simulink model "hodumaru"  (R2023a)
settings: Solver=VariableStepAuto  StartTime=0.0  StopTime=10.0  RelTol=1e-3
undefined symbols (not defined in the file): _NA, Addr, Control, DFSW, DSFW, Kill, NeuralCodedData, R_EN, RC, RC_FINAL, Spike
(part 1 of 2)
settings Model: Creator=user  LastModifiedBy=x1t2

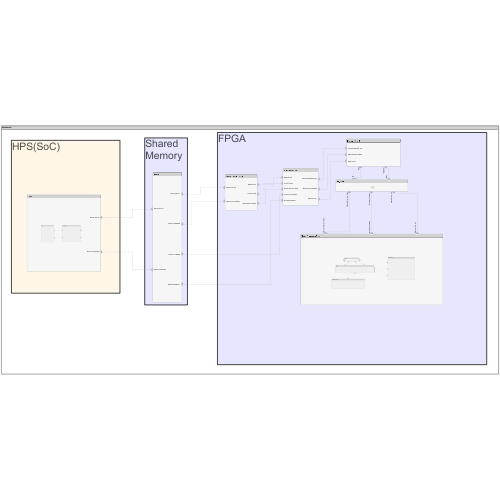
[thumbnail: Simulink's stored preview of the top-level diagram]
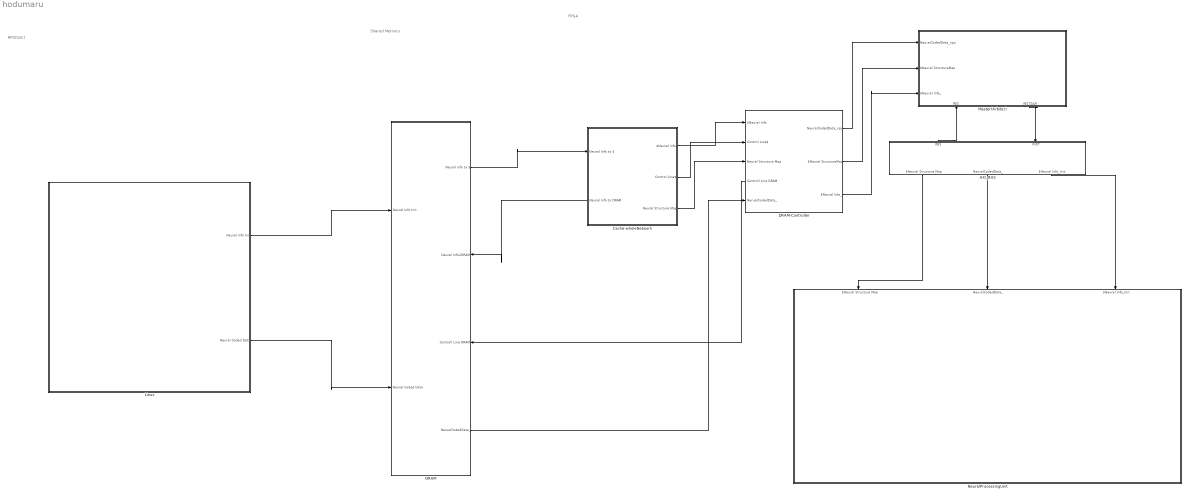
== system hodumaru ==
  note: Shared
      | Memory
  note: HPS(SoC)
  note: FPGA
  AXI_BUS : Subsystem
      settings: PortSchema="{\"entries\":[{\"content\":{\"headerSize\":26,\"margin\":15,\"minimumSpacing\":25,\"sides\":[{\"content\":{},\"type\":\"ConnectorPlacement.EquallySpacedRectSide\",\"uuid\":\"08b5c2e0-5e4b-4108-9213-5cb3cfbc2fc7\"},{\"content\":{\"side\":\"RIGHT\"},\"type\":\"ConnectorPlacement.EquallySpacedRectSide\",\"uuid\":\"cef344b6-f3e5-417a-912f-da0044eb54ca\"},{\"content\":{\"connectorIds\":[\"Out3\",\"In1\"],\"side\":\"TOP\"},\"type\":\"ConnectorPlacement.EquallySpacedRectSide\",\"uuid\":\"0b83641f-e918-4d2c-8db0-09bb563129af\"},{\"content\":{\"connectorIds\":[\"Out1\",\"Out2\",\"Out4\"],\"side\":\"BOTTOM\"},\"type\":\"ConnectorPlacement.EquallySpacedRectSide\",\"uuid\":\"7ad7297b-5e88-44bc-b04f-1700d4001bfc\"}]},\"type\":\"ConnectorPlacement.EquallySpacedConnector\",\"uuid\":\"45bfd962-fc80-412c-925f-742c48c6b5c0\"}],\"packageUris\":[\"http://schema.mathworks.com/mf0/Connector/R2020b\"],\"version\":\"1.0\"}"
  Cache-wholeNetwork : Subsystem
      settings: PortSchema="{\"entries\":[{\"content\":{\"headerSize\":26,\"margin\":15,\"minimumSpacing\":25,\"sides\":[{\"content\":{\"connectorIds\":[\"In1\",\"Out4\"]},\"type\":\"ConnectorPlacement.EquallySpacedRectSide\",\"uuid\":\"08b5c2e0-5e4b-4108-9213-5cb3cfbc2fc7\"},{\"content\":{\"connectorIds\":[\"Out2\",\"Out3\",\"Out1\"],\"side\":\"RIGHT\"},\"type\":\"ConnectorPlacement.EquallySpacedRectSide\",\"uuid\":\"cef344b6-f3e5-417a-912f-da0044eb54ca\"},{\"content\":{\"side\":\"TOP\"},\"type\":\"ConnectorPlacement.EquallySpacedRectSide\",\"uuid\":\"0b83641f-e918-4d2c-8db0-09bb563129af\"},{\"content\":{\"side\":\"BOTTOM\"},\"type\":\"ConnectorPlacement.EquallySpacedRectSide\",\"uuid\":\"59b98d3e-8ece-4a5f-b745-8d3a946f67db\"}]},\"type\":\"ConnectorPlacement.EquallySpacedConnector\",\"uuid\":\"45bfd962-fc80-412c-925f-742c48c6b5c0\"}],\"packageUris\":[\"http://schema.mathworks.com/mf0/Connector/R2020b\"],\"version\":\"1.0\"}"
  DRAM : Subsystem
      settings: PortSchema="{\"entries\":[{\"content\":{\"headerSize\":26,\"margin\":15,\"minimumSpacing\":25,\"sides\":[{\"content\":{\"connectorIds\":[\"In1\",\"In2\"]},\"type\":\"ConnectorPlacement.EquallySpacedRectSide\",\"uuid\":\"08b5c2e0-5e4b-4108-9213-5cb3cfbc2fc7\"},{\"content\":{\"connectorIds\":[\"Out1\",\"In4\",\"In3\",\"Out2\"],\"side\":\"RIGHT\"},\"type\":\"ConnectorPlacement.EquallySpacedRectSide\",\"uuid\":\"cef344b6-f3e5-417a-912f-da0044eb54ca\"},{\"content\":{\"side\":\"TOP\"},\"type\":\"ConnectorPlacement.EquallySpacedRectSide\",\"uuid\":\"0b83641f-e918-4d2c-8db0-09bb563129af\"}]},\"type\":\"ConnectorPlacement.EquallySpacedConnector\",\"uuid\":\"45bfd962-fc80-412c-925f-742c48c6b5c0\"}],\"packageUris\":[\"http://schema.mathworks.com/mf0/Connector/R2020b\"],\"version\":\"1.0\"}"
  DRAM-Controller : Subsystem
      settings: PortSchema="{\"entries\":[{\"content\":{\"headerSize\":26,\"margin\":15,\"minimumSpacing\":25,\"sides\":[{\"content\":{\"connectorIds\":[\"In1\",\"In2\",\"In3\",\"Out1\",\"In4\"]},\"type\":\"ConnectorPlacement.EquallySpacedRectSide\",\"uuid\":\"08b5c2e0-5e4b-4108-9213-5cb3cfbc2fc7\"},{\"content\":{\"connectorIds\":[\"Out3\",\"Out2\",\"Out4\"],\"side\":\"RIGHT\"},\"type\":\"ConnectorPlacement.EquallySpacedRectSide\",\"uuid\":\"cef344b6-f3e5-417a-912f-da0044eb54ca\"},{\"content\":{\"side\":\"TOP\"},\"type\":\"ConnectorPlacement.EquallySpacedRectSide\",\"uuid\":\"0b83641f-e918-4d2c-8db0-09bb563129af\"},{\"content\":{\"side\":\"BOTTOM\"},\"type\":\"ConnectorPlacement.EquallySpacedRectSide\",\"uuid\":\"f4226d07-ea44-47f7-aa94-5b35827b4c18\"}]},\"type\":\"ConnectorPlacement.EquallySpacedConnector\",\"uuid\":\"45bfd962-fc80-412c-925f-742c48c6b5c0\"}],\"packageUris\":[\"http://schema.mathworks.com/mf0/Connector/R2020b\"],\"version\":\"1.0\"}"
  Linux : Subsystem
      settings: PortSchema="{\"entries\":[{\"content\":{\"headerSize\":26,\"margin\":15,\"minimumSpacing\":25,\"sides\":[{\"content\":{},\"type\":\"ConnectorPlacement.EquallySpacedRectSide\",\"uuid\":\"31e20200-2cb1-4382-9155-e0d85eeb6756\"},{\"content\":{\"connectorIds\":[\"Out1\",\"Out2\"],\"side\":\"RIGHT\"},\"type\":\"ConnectorPlacement.EquallySpacedRectSide\",\"uuid\":\"e7a9e024-b9ad-4463-a43b-85143ff39b21\"},{\"content\":{\"side\":\"TOP\"},\"type\":\"ConnectorPlacement.EquallySpacedRectSide\",\"uuid\":\"8c8eb66f-8faf-4222-8ab7-6c33983befa5\"}]},\"type\":\"ConnectorPlacement.EquallySpacedConnector\",\"uuid\":\"7102759c-7f33-40ec-8288-a87a26b0547f\"}],\"packageUris\":[\"http://schema.mathworks.com/mf0/Connector/R2020b\"],\"version\":\"1.0\"}"
  Master(Arbiter) : Subsystem
      settings: PortSchema="{\"entries\":[{\"content\":{\"headerSize\":26,\"margin\":15,\"minimumSpacing\":25,\"sides\":[{\"content\":{\"connectorIds\":[\"In1\",\"In2\",\"In3\"]},\"type\":\"ConnectorPlacement.EquallySpacedRectSide\",\"uuid\":\"08b5c2e0-5e4b-4108-9213-5cb3cfbc2fc7\"},{\"content\":{\"side\":\"RIGHT\"},\"type\":\"ConnectorPlacement.EquallySpacedRectSide\",\"uuid\":\"cef344b6-f3e5-417a-912f-da0044eb54ca\"},{\"content\":{\"side\":\"TOP\"},\"type\":\"ConnectorPlacement.EquallySpacedRectSide\",\"uuid\":\"0b83641f-e918-4d2c-8db0-09bb563129af\"},{\"content\":{\"connectorIds\":[\"In4\",\"Out1\"],\"side\":\"BOTTOM\"},\"type\":\"ConnectorPlacement.EquallySpacedRectSide\",\"uuid\":\"f397b488-8c38-49a3-8091-fc0d0544b256\"}]},\"type\":\"ConnectorPlacement.EquallySpacedConnector\",\"uuid\":\"45bfd962-fc80-412c-925f-742c48c6b5c0\"}],\"packageUris\":[\"http://schema.mathworks.com/mf0/Connector/R2020b\"],\"version\":\"1.0\"}"
  NeuralProcessingUnit : Subsystem
      settings: PortSchema="{\"entries\":[{\"content\":{\"headerSize\":26,\"margin\":15,\"minimumSpacing\":25,\"sides\":[{\"content\":{},\"type\":\"ConnectorPlacement.EquallySpacedRectSide\",\"uuid\":\"08b5c2e0-5e4b-4108-9213-5cb3cfbc2fc7\"},{\"content\":{\"side\":\"RIGHT\"},\"type\":\"ConnectorPlacement.EquallySpacedRectSide\",\"uuid\":\"cef344b6-f3e5-417a-912f-da0044eb54ca\"},{\"content\":{\"connectorIds\":[\"In1\",\"In2\",\"In3\"],\"side\":\"TOP\"},\"type\":\"ConnectorPlacement.EquallySpacedRectSide\",\"uuid\":\"0b83641f-e918-4d2c-8db0-09bb563129af\"},{\"content\":{\"side\":\"BOTTOM\"},\"type\":\"ConnectorPlacement.EquallySpacedRectSide\",\"uuid\":\"28924508-1ca7-4062-8931-456146d3b2a8\"}]},\"type\":\"ConnectorPlacement.EquallySpacedConnector\",\"uuid\":\"45bfd962-fc80-412c-925f-742c48c6b5c0\"}],\"packageUris\":[\"http://schema.mathworks.com/mf0/Connector/R2020b\"],\"version\":\"1.0\"}"
  wires:
  Master(Arbiter)/1(INST2AXI) -> AXI_BUS/1(INST)
  AXI_BUS/3(RES) -> Master(Arbiter)/4(RES)
  Cache-wholeNetwork/2($Neural Info) -> DRAM-Controller/1($Neural Info)
  DRAM-Controller/4($Neural Info_) -> Master(Arbiter)/3($Neural Info_)
  DRAM/1(Neural Info to $) -> Cache-wholeNetwork/1(Neural Info to $)
  Cache-wholeNetwork/4(Neural Info to DRAM) -> DRAM/4(Neural Info2DRAM)
  Cache-wholeNetwork/3(Control Line$) -> DRAM-Controller/2(Control Line$)
  DRAM-Controller/1(Controll Line DRAM) -> DRAM/3(Controll Line DRAM)
  AXI_BUS/4($Neural Info_Init) -> NeuralProcessingUnit/3($Neural Info_Init)
  Linux/2(Neural Coded Data) -> DRAM/2(Neural Coded Data)
  DRAM/2(NerualCodedData_) -> DRAM-Controller/4(NerualCodedData_)
  DRAM-Controller/3(NeuralCodedData_npu) -> Master(Arbiter)/1(NeuralCodedData_npu)
  AXI_BUS/2(NeuralCodedData_) -> NeuralProcessingUnit/2(NeuralCodedData_)
  Cache-wholeNetwork/1(Neural Structure Map) -> DRAM-Controller/3(Neural Structure Map)
  DRAM-Controller/2($Neural StructureMap) -> Master(Arbiter)/2($Neural StructureMap)
  AXI_BUS/1($Neural Structure Map) -> NeuralProcessingUnit/1($Neural Structure Map)
  Linux/1(Neural Info Init) -> DRAM/1(Neural Info Init)

== system hodumaru/AXI_BUS ==
  Bus Element In3 : Inport  PortName=INST
  Component : Subsystem
      settings: PortSchema="{\"entries\":[{\"content\":{\"headerSize\":26,\"margin\":15,\"minimumSpacing\":25,\"sides\":[{\"content\":{},\"type\":\"ConnectorPlacement.EquallySpacedRectSide\",\"uuid\":\"514d6b75-8d61-4949-8a22-d0c879126762\"},{\"content\":{\"side\":\"RIGHT\"},\"type\":\"ConnectorPlacement.EquallySpacedRectSide\",\"uuid\":\"7fd721c4-6b30-4b2e-9e28-1df8eaa236c6\"},{\"content\":{\"side\":\"TOP\"},\"type\":\"ConnectorPlacement.EquallySpacedRectSide\",\"uuid\":\"aef488b6-1070-4811-8456-2792a187eb4f\"},{\"content\":{\"connectorIds\":[\"Out1\",\"In1\"],\"side\":\"BOTTOM\"},\"type\":\"ConnectorPlacement.EquallySpacedRectSide\",\"uuid\":\"0b4565ad-3b23-437a-a747-07b7ba558033\"}]},\"type\":\"ConnectorPlacement.EquallySpacedConnector\",\"uuid\":\"39ef6a1a-935b-4f2a-a1aa-febde07ec6b8\"}],\"packageUris\":[\"http://schema.mathworks.com/mf0/Connector/R2020b\"],\"version\":\"1.0\"}"
  Bus Element Out1 : Outport  PortName=$Neural Structure Map
  Bus Element Out4 : Outport  Port=2  PortName=NeuralCodedData_
  Bus Element Out2 : Outport  Port=3  PortName=RES
  Bus Element Out3 : Outport  Port=4  PortName=$Neural Info_Init
  wires:
  Component/1(RES) -> Bus Element Out2/1
  ? -> Component/1($PARAM2AXI)

== system hodumaru/Cache-wholeNetwork ==
  Bus Element In2 : Inport  PortName=Neural Info to $
  Bus Element Out4 : Outport  PortName=Neural Structure Map
  Bus Element Out2 : Outport  Port=2  PortName=$Neural Info
  Bus Element Out3 : Outport  Port=3  PortName=Control Line$
  Bus Element Out1 : Outport  Port=4  PortName=Neural Info to DRAM

== system hodumaru/DRAM ==
  Bus Element In4 : Inport  PortName=Neural Info Init
  Bus Element In3 : Inport  Port=2  PortName=Neural Coded Data
  Bus Element In2 : Inport  Port=3  PortName=Controll Line DRAM
  Bus Element In1 : Inport  Port=4  PortName=Neural Info2DRAM
  Bus Element Out3 : Outport  PortName=Neural Info to $
  Bus Element Out2 : Outport  Port=2  PortName=NerualCodedData_

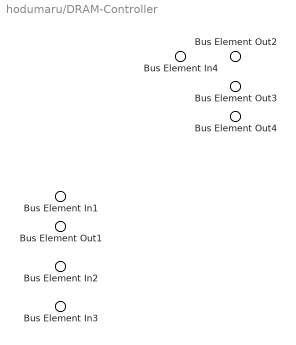
== system hodumaru/DRAM-Controller ==
  Bus Element In1 : Inport  PortName=$Neural Info
  Bus Element In2 : Inport  Port=2  PortName=Control Line$
  Bus Element In4 : Inport  Port=3  PortName=Neural Structure Map
  Bus Element In3 : Inport  Port=4  PortName=NerualCodedData_
  Bus Element Out2 : Outport  PortName=Controll Line DRAM
  Bus Element Out4 : Outport  Port=2  PortName=$Neural StructureMap
  Bus Element Out3 : Outport  Port=3  PortName=NeuralCodedData_npu
  Bus Element Out1 : Outport  Port=4  PortName=$Neural Info_

== system hodumaru/Linux ==
  Input Data : Subsystem
      settings: PortSchema="{\"entries\":[{\"content\":{\"headerSize\":26,\"margin\":15,\"minimumSpacing\":25,\"sides\":[{\"content\":{},\"type\":\"ConnectorPlacement.EquallySpacedRectSide\",\"uuid\":\"31e20200-2cb1-4382-9155-e0d85eeb6756\"},{\"content\":{\"connectorIds\":[\"Out1\",\"Out2\"],\"side\":\"RIGHT\"},\"type\":\"ConnectorPlacement.EquallySpacedRectSide\",\"uuid\":\"e7a9e024-b9ad-4463-a43b-85143ff39b21\"},{\"content\":{\"side\":\"TOP\"},\"type\":\"ConnectorPlacement.EquallySpacedRectSide\",\"uuid\":\"8c8eb66f-8faf-4222-8ab7-6c33983befa5\"}]},\"type\":\"ConnectorPlacement.EquallySpacedConnector\",\"uuid\":\"7102759c-7f33-40ec-8288-a87a26b0547f\"}],\"packageUris\":[\"http://schema.mathworks.com/mf0/Connector/R2020b\"],\"version\":\"1.0\"}"
  Neural Coding Engine : Subsystem
      settings: PortSchema="{\"entries\":[{\"content\":{\"headerSize\":26,\"margin\":15,\"minimumSpacing\":25,\"sides\":[{\"content\":{\"connectorIds\":[\"In1\",\"In2\"]},\"type\":\"ConnectorPlacement.EquallySpacedRectSide\",\"uuid\":\"31e20200-2cb1-4382-9155-e0d85eeb6756\"},{\"content\":{\"connectorIds\":[\"Out1\",\"Out2\"],\"side\":\"RIGHT\"},\"type\":\"ConnectorPlacement.EquallySpacedRectSide\",\"uuid\":\"e7a9e024-b9ad-4463-a43b-85143ff39b21\"},{\"content\":{\"side\":\"TOP\"},\"type\":\"ConnectorPlacement.EquallySpacedRectSide\",\"uuid\":\"8c8eb66f-8faf-4222-8ab7-6c33983befa5\"}]},\"type\":\"ConnectorPlacement.EquallySpacedConnector\",\"uuid\":\"7102759c-7f33-40ec-8288-a87a26b0547f\"}],\"packageUris\":[\"http://schema.mathworks.com/mf0/Connector/R2020b\"],\"version\":\"1.0\"}"
  Bus Element Out2 : Outport  PortName=Neural Info Init
  Bus Element Out1 : Outport  Port=2  PortName=Neural Coded Data
  wires:
  Input Data/2(DATA) -> Neural Coding Engine/2(DATA)
  Neural Coding Engine/2(Neural Coded Data) -> Bus Element Out1/1
  Input Data/1(Neural Info Init) -> Neural Coding Engine/1(Neural Info Init)
  Neural Coding Engine/1(OutBus) -> Bus Element Out2/1

== system hodumaru/Master(Arbiter) ==
  Bus Element In2 : Inport  PortName=NeuralCodedData_npu
  Bus Element In4 : Inport  Port=2  PortName=$Neural StructureMap
  Bus Element In3 : Inport  Port=3  PortName=$Neural Info_
  Bus Element In1 : Inport  Port=4  PortName=RES
  Bus Element Out1 : Outport  PortName=INST2AXI

== system hodumaru/NeuralProcessingUnit ==
  Bus Element In2 : Inport  PortName=$Neural Structure Map
  Bus Element In3 : Inport  Port=2  PortName=NeuralCodedData_
  Bus Element In1 : Inport  Port=3  PortName=$Neural Info_Init
  AXIBus : Subsystem
      settings: PortSchema="{\"entries\":[{\"content\":{\"headerSize\":26,\"margin\":15,\"minimumSpacing\":25,\"sides\":[{\"content\":{},\"type\":\"ConnectorPlacement.EquallySpacedRectSide\",\"uuid\":\"08b5c2e0-5e4b-4108-9213-5cb3cfbc2fc7\"},{\"content\":{\"connectorIds\":[\"Out2\",\"In2\",\"Out3\"],\"side\":\"RIGHT\"},\"type\":\"ConnectorPlacement.EquallySpacedRectSide\",\"uuid\":\"cef344b6-f3e5-417a-912f-da0044eb54ca\"},{\"content\":{\"connectorIds\":[\"In1\",\"Out4\"],\"side\":\"TOP\"},\"type\":\"ConnectorPlacement.EquallySpacedRectSide\",\"uuid\":\"0b83641f-e918-4d2c-8db0-09bb563129af\"},{\"content\":{\"connectorIds\":[\"Out1\"],\"side\":\"BOTTOM\"},\"type\":\"ConnectorPlacement.EquallySpacedRectSide\",\"uuid\":\"b9d6ab38-6789-4ab1-ad47-3b4db5a60e34\"}]},\"type\":\"ConnectorPlacement.EquallySpacedConnector\",\"uuid\":\"45bfd962-fc80-412c-925f-742c48c6b5c0\"}],\"packageUris\":[\"http://schema.mathworks.com/mf0/Connector/R2020b\"],\"version\":\"1.0\"}"
  MC Connection Cache : Subsystem
      settings: PortSchema="{\"entries\":[{\"content\":{\"headerSize\":26,\"margin\":15,\"minimumSpacing\":25,\"sides\":[{\"content\":{},\"type\":\"ConnectorPlacement.EquallySpacedRectSide\",\"uuid\":\"31e20200-2cb1-4382-9155-e0d85eeb6756\"},{\"content\":{\"side\":\"RIGHT\"},\"type\":\"ConnectorPlacement.EquallySpacedRectSide\",\"uuid\":\"e7a9e024-b9ad-4463-a43b-85143ff39b21\"},{\"content\":{\"connectorIds\":[\"In1\"],\"side\":\"TOP\"},\"type\":\"ConnectorPlacement.EquallySpacedRectSide\",\"uuid\":\"8c8eb66f-8faf-4222-8ab7-6c33983befa5\"}]},\"type\":\"ConnectorPlacement.EquallySpacedConnector\",\"uuid\":\"7102759c-7f33-40ec-8288-a87a26b0547f\"}],\"packageUris\":[\"http://schema.mathworks.com/mf0/Connector/R2020b\"],\"version\":\"1.0\"}"
  Master : Subsystem
      settings: PortSchema="{\"entries\":[{\"content\":{\"headerSize\":26,\"margin\":15,\"minimumSpacing\":25,\"sides\":[{\"content\":{\"connectorIds\":[\"In1\",\"In2\"]},\"type\":\"ConnectorPlacement.EquallySpacedRectSide\",\"uuid\":\"08b5c2e0-5e4b-4108-9213-5cb3cfbc2fc7\"},{\"content\":{\"connectorIds\":[\"In3\"],\"side\":\"RIGHT\"},\"type\":\"ConnectorPlacement.EquallySpacedRectSide\",\"uuid\":\"cef344b6-f3e5-417a-912f-da0044eb54ca\"},{\"content\":{\"side\":\"TOP\"},\"type\":\"ConnectorPlacement.EquallySpacedRectSide\",\"uuid\":\"0b83641f-e918-4d2c-8db0-09bb563129af\"},{\"content\":{\"connectorIds\":[\"Out1\",\"In4\"],\"side\":\"BOTTOM\"},\"type\":\"ConnectorPlacement.EquallySpacedRectSide\",\"uuid\":\"dc121f09-b3e7-47bb-989d-1802dc981a21\"}]},\"type\":\"ConnectorPlacement.EquallySpacedConnector\",\"uuid\":\"45bfd962-fc80-412c-925f-742c48c6b5c0\"}],\"packageUris\":[\"http://schema.mathworks.com/mf0/Connector/R2020b\"],\"version\":\"1.0\"}"
  MiniColumn(Array) : Subsystem
      settings: PortSchema="{\"entries\":[{\"content\":{\"headerSize\":26,\"margin\":15,\"minimumSpacing\":25,\"sides\":[{\"content\":{\"connectorIds\":[\"In1\",\"Out1\",\"In2\"]},\"type\":\"ConnectorPlacement.EquallySpacedRectSide\",\"uuid\":\"08b5c2e0-5e4b-4108-9213-5cb3cfbc2fc7\"},{\"content\":{\"side\":\"RIGHT\"},\"type\":\"ConnectorPlacement.EquallySpacedRectSide\",\"uuid\":\"cef344b6-f3e5-417a-912f-da0044eb54ca\"},{\"content\":{\"side\":\"TOP\"},\"type\":\"ConnectorPlacement.EquallySpacedRectSide\",\"uuid\":\"0b83641f-e918-4d2c-8db0-09bb563129af\"},{\"content\":{\"side\":\"BOTTOM\"},\"type\":\"ConnectorPlacement.EquallySpacedRectSide\",\"uuid\":\"558f9d34-057e-41c8-af81-9bce1d5389a5\"}]},\"type\":\"ConnectorPlacement.EquallySpacedConnector\",\"uuid\":\"45bfd962-fc80-412c-925f-742c48c6b5c0\"}],\"packageUris\":[\"http://schema.mathworks.com/mf0/Connector/R2020b\"],\"version\":\"1.0\"}"
  wires:
  MiniColumn(Array)/1(OutBus) -> AXIBus/2(InBus)
  Master/1(OutBus) -> AXIBus/1(InBus1)
  AXIBus/4(OutBus1) -> Master/4(InBus)
  Bus Element In1/1 -> Master/3($Neural Info_Init)
  AXIBus/2($Neural Info Init_) -> MiniColumn(Array)/1($Neural Info Init_)
  Bus Element In3/1 -> Master/2(NeuralCodedData_)
  AXIBus/3(NeuralCodedData_MC) -> MiniColumn(Array)/2(NeuralCodedData_MC)
  Bus Element In2/1 -> Master/1($Neural Structure Map)
  AXIBus/1(Neural Structure Map) -> MC Connection Cache/1(Neural Structure Map)

== system hodumaru/AXI_BUS/Component ==
  Bus Element In1 : Inport  PortName=$PARAM2AXI
  Bus Element Out1 : Outport  PortName=RES

== system hodumaru/Linux/Input Data ==
  Bus Element Out2 : Outport  PortName=Neural Info Init
  Bus Element Out1 : Outport  Port=2  PortName=DATA

== system hodumaru/Linux/Neural Coding Engine ==
  Bus Element In2 : Inport  PortName=Neural Info Init
  Bus Element In1 : Inport  Port=2  PortName=DATA
  Bus Element Out2 : Outport  PortName=OutBus
  Bus Element Out1 : Outport  Port=2  PortName=Neural Coded Data

== system hodumaru/NeuralProcessingUnit/AXIBus ==
  Bus Element In3 : Inport  PortName=InBus1
  Bus Element In2 : Inport  Port=2  PortName=InBus
  Bus Element Out1 : Outport  PortName=Neural Structure Map
  Bus Element Out2 : Outport  Port=2  PortName=$Neural Info Init_
  Bus Element Out4 : Outport  Port=3  PortName=NeuralCodedData_MC
  Bus Element Out3 : Outport  Port=4  PortName=OutBus1

== system hodumaru/NeuralProcessingUnit/MC Connection Cache ==
  Bus Element In1 : Inport  PortName=Neural Structure Map

== system hodumaru/NeuralProcessingUnit/Master ==
  Bus Element In4 : Inport  PortName=$Neural Structure Map
  Bus Element In3 : Inport  Port=2  PortName=NeuralCodedData_
  Bus Element In2 : Inport  Port=3  PortName=$Neural Info_Init
  Bus Element In1 : Inport  Port=4  PortName=InBus
  Bus Element Out1 : Outport  PortName=OutBus

== system hodumaru/NeuralProcessingUnit/MiniColumn(Array) ==
  Bus Element In2 : Inport  PortName=$Neural Info Init_
  Bus Element In3 : Inport  Port=2  PortName=NeuralCodedData_MC
  AXIBus : Subsystem
      settings: PortSchema="{\"entries\":[{\"content\":{\"headerSize\":26,\"margin\":15,\"minimumSpacing\":25,\"sides\":[{\"content\":{\"connectorIds\":[\"In1\",\"In2\"]},\"type\":\"ConnectorPlacement.EquallySpacedRectSide\",\"uuid\":\"08b5c2e0-5e4b-4108-9213-5cb3cfbc2fc7\"},{\"content\":{\"connectorIds\":[\"In4\",\"Out6\"],\"side\":\"RIGHT\"},\"type\":\"ConnectorPlacement.EquallySpacedRectSide\",\"uuid\":\"cef344b6-f3e5-417a-912f-da0044eb54ca\"},{\"content\":{\"side\":\"TOP\"},\"type\":\"ConnectorPlacement.EquallySpacedRectSide\",\"uuid\":\"0b83641f-e918-4d2c-8db0-09bb563129af\"},{\"content\":{\"connectorIds\":[\"Out7\",\"Out1\",\"In3\",\"Out2\",\"Out3\",\"Out4\",\"In5\",\"Out5\"],\"side\":\"BOTTOM\"},\"type\":\"ConnectorPlacement.EquallySpacedRectSide\",\"uuid\":\"063ff189-0b4f-497b-a1fa-91bf1e0a9e70\"}]},\"type\":\"ConnectorPlacement.EquallySpacedConnector\",\"uuid\":\"45bfd962-fc80-412c-925f-742c48c6b5c0\"}],\"packageUris\":[\"http://schema.mathworks.com/mf0/Connector/R2020b\"],\"version\":\"1.0\"}"
  MiniColumn1 : Subsystem
      settings: PortSchema="{\"entries\":[{\"content\":{\"headerSize\":26,\"margin\":15,\"minimumSpacing\":25,\"sides\":[{\"content\":{},\"type\":\"ConnectorPlacement.EquallySpacedRectSide\",\"uuid\":\"08b5c2e0-5e4b-4108-9213-5cb3cfbc2fc7\"},{\"content\":{\"side\":\"RIGHT\"},\"type\":\"ConnectorPlacement.EquallySpacedRectSide\",\"uuid\":\"cef344b6-f3e5-417a-912f-da0044eb54ca\"},{\"content\":{\"connectorIds\":[\"In1\",\"In2\",\"Out2\",\"In3\"],\"side\":\"TOP\"},\"type\":\"ConnectorPlacement.EquallySpacedRectSide\",\"uuid\":\"0b83641f-e918-4d2c-8db0-09bb563129af\"},{\"content\":{\"connectorIds\":[\"Out1\"],\"side\":\"BOTTOM\"},\"type\":\"ConnectorPlacement.EquallySpacedRectSide\",\"uuid\":\"32b006f9-ec9b-4081-80fb-80d6b64b9ab2\"}]},\"type\":\"ConnectorPlacement.EquallySpacedConnector\",\"uuid\":\"45bfd962-fc80-412c-925f-742c48c6b5c0\"}],\"packageUris\":[\"http://schema.mathworks.com/mf0/Connector/R2020b\"],\"version\":\"1.0\"}"
  MiniColumn2 : Subsystem
      settings: PortSchema="{\"entries\":[{\"content\":{\"headerSize\":26,\"margin\":15,\"minimumSpacing\":25,\"sides\":[{\"content\":{},\"type\":\"ConnectorPlacement.EquallySpacedRectSide\",\"uuid\":\"08b5c2e0-5e4b-4108-9213-5cb3cfbc2fc7\"},{\"content\":{\"side\":\"RIGHT\"},\"type\":\"ConnectorPlacement.EquallySpacedRectSide\",\"uuid\":\"cef344b6-f3e5-417a-912f-da0044eb54ca\"},{\"content\":{\"connectorIds\":[\"In1\",\"In2\",\"Out2\",\"In3\"],\"side\":\"TOP\"},\"type\":\"ConnectorPlacement.EquallySpacedRectSide\",\"uuid\":\"0b83641f-e918-4d2c-8db0-09bb563129af\"},{\"content\":{\"connectorIds\":[\"Out1\"],\"side\":\"BOTTOM\"},\"type\":\"ConnectorPlacement.EquallySpacedRectSide\",\"uuid\":\"32b006f9-ec9b-4081-80fb-80d6b64b9ab2\"}]},\"type\":\"ConnectorPlacement.EquallySpacedConnector\",\"uuid\":\"45bfd962-fc80-412c-925f-742c48c6b5c0\"}],\"packageUris\":[\"http://schema.mathworks.com/mf0/Connector/R2020b\"],\"version\":\"1.0\"}"
  RichClubMemory(MCNI) : Subsystem
      settings: PortSchema="{\"entries\":[{\"content\":{\"headerSize\":26,\"margin\":15,\"minimumSpacing\":25,\"sides\":[{\"content\":{\"connectorIds\":[\"Out1\",\"In1\"]},\"type\":\"ConnectorPlacement.EquallySpacedRectSide\",\"uuid\":\"08b5c2e0-5e4b-4108-9213-5cb3cfbc2fc7\"},{\"content\":{\"side\":\"RIGHT\"},\"type\":\"ConnectorPlacement.EquallySpacedRectSide\",\"uuid\":\"cef344b6-f3e5-417a-912f-da0044eb54ca\"},{\"content\":{\"side\":\"TOP\"},\"type\":\"ConnectorPlacement.EquallySpacedRectSide\",\"uuid\":\"0b83641f-e918-4d2c-8db0-09bb563129af\"}]},\"type\":\"ConnectorPlacement.EquallySpacedConnector\",\"uuid\":\"45bfd962-fc80-412c-925f-742c48c6b5c0\"}],\"packageUris\":[\"http://schema.mathworks.com/mf0/Connector/R2020b\"],\"version\":\"1.0\"}"
  Bus Element Out1 : Outport  PortName=OutBus
  wires:
  MiniColumn1/2(RC PostSpiketoOuter) -> AXIBus/5(RC PostSpiketoOuter1)
  AXIBus/7(RC PoskSpike From another MC1) -> MiniColumn2/1(RC PoskSpike From another MC)
  AXIBus/6(OutBus) -> RichClubMemory(MCNI)/1(InBus)
  RichClubMemory(MCNI)/1(OutBus) -> AXIBus/4(InBus1)
  AXIBus/5($Neural Info Init_MC1) -> MiniColumn1/3($Neural Info Init_MC)
  AXIBus/4(NeuralCodedData1) -> MiniColumn1/2(NeuralCodedData)
  AXIBus/1(NeuralCodedData) -> MiniColumn2/2(NeuralCodedData)
  MiniColumn2/2(RC PostSpiketoOuter) -> AXIBus/3(RC PostSpiketoOuter)
  AXIBus/2($Neural Info Init_MC) -> MiniColumn2/3($Neural Info Init_MC)
  AXIBus/3(RC PostSpike From Another MC2) -> MiniColumn1/1(RC PostSpike From Another MC2)
  Bus Element In3/1 -> AXIBus/2(NeuralCodedData_MC)
  Bus Element In2/1 -> AXIBus/1($Neural Info Init_)

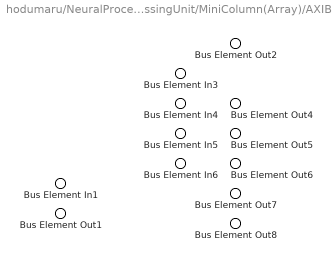
== system hodumaru/NeuralProcessingUnit/MiniColumn(Array)/AXIBus ==
  Bus Element In6 : Inport  PortName=$Neural Info Init_
  Bus Element In5 : Inport  Port=2  PortName=NeuralCodedData_MC
  Bus Element In4 : Inport  Port=3  PortName=RC PostSpiketoOuter
  Bus Element In3 : Inport  Port=4  PortName=InBus1
  Bus Element In1 : Inport  Port=5  PortName=RC PostSpiketoOuter1
  Bus Element Out6 : Outport  PortName=NeuralCodedData
  Bus Element Out7 : Outport  Port=2  PortName=$Neural Info Init_MC
  Bus Element Out8 : Outport  Port=3  PortName=RC PostSpike From Another MC2
  Bus Element Out5 : Outport  Port=4  PortName=NeuralCodedData1
  Bus Element Out4 : Outport  Port=5  PortName=$Neural Info Init_MC1
  Bus Element Out2 : Outport  Port=6  PortName=OutBus
  Bus Element Out1 : Outport  Port=7  PortName=RC PoskSpike From another MC1

== system hodumaru/NeuralProcessingUnit/MiniColumn(Array)/MiniColumn1 ==
  Bus Element In3 : Inport  PortName=RC PostSpike From Another MC2
  Bus Element In2 : Inport  Port=2  PortName=NeuralCodedData
  Bus Element In1 : Inport  Port=3  PortName=$Neural Info Init_MC
  AXIBus : Subsystem
      settings: PortSchema="{\"entries\":[{\"content\":{\"headerSize\":26,\"margin\":15,\"minimumSpacing\":25,\"sides\":[{\"content\":{},\"type\":\"ConnectorPlacement.EquallySpacedRectSide\",\"uuid\":\"08b5c2e0-5e4b-4108-9213-5cb3cfbc2fc7\"},{\"content\":{\"connectorIds\":[\"Out4\",\"Out5\"],\"side\":\"RIGHT\"},\"type\":\"ConnectorPlacement.EquallySpacedRectSide\",\"uuid\":\"cef344b6-f3e5-417a-912f-da0044eb54ca\"},{\"content\":{\"connectorIds\":[\"In1\",\"Out3\"],\"side\":\"TOP\"},\"type\":\"ConnectorPlacement.EquallySpacedRectSide\",\"uuid\":\"0b83641f-e918-4d2c-8db0-09bb563129af\"},{\"content\":{\"connectorIds\":[\"Out1\",\"Out2\",\"In2\",\"In3\",\"In4\"],\"side\":\"BOTTOM\"},\"type\":\"ConnectorPlacement.EquallySpacedRectSide\",\"uuid\":\"19498b06-f260-4dc1-a094-027c00d8d906\"}]},\"type\":\"ConnectorPlacement.EquallySpacedConnector\",\"uuid\":\"45bfd962-fc80-412c-925f-742c48c6b5c0\"}],\"packageUris\":[\"http://schema.mathworks.com/mf0/Connector/R2020b\"],\"version\":\"1.0\"}"
  MAster : Subsystem
      settings: PortSchema="{\"entries\":[{\"content\":{\"headerSize\":26,\"margin\":15,\"minimumSpacing\":25,\"sides\":[{\"content\":{\"connectorIds\":[\"In1\",\"In2\"]},\"type\":\"ConnectorPlacement.EquallySpacedRectSide\",\"uuid\":\"08b5c2e0-5e4b-4108-9213-5cb3cfbc2fc7\"},{\"content\":{\"connectorIds\":[\"In3\"],\"side\":\"RIGHT\"},\"type\":\"ConnectorPlacement.EquallySpacedRectSide\",\"uuid\":\"cef344b6-f3e5-417a-912f-da0044eb54ca\"},{\"content\":{\"side\":\"TOP\"},\"type\":\"ConnectorPlacement.EquallySpacedRectSide\",\"uuid\":\"0b83641f-e918-4d2c-8db0-09bb563129af\"},{\"content\":{\"connectorIds\":[\"Out1\",\"In4\"],\"side\":\"BOTTOM\"},\"type\":\"ConnectorPlacement.EquallySpacedRectSide\",\"uuid\":\"1d0526f4-c594-4b80-8124-d3d48d90ce30\"}]},\"type\":\"ConnectorPlacement.EquallySpacedConnector\",\"uuid\":\"45bfd962-fc80-412c-925f-742c48c6b5c0\"}],\"packageUris\":[\"http://schema.mathworks.com/mf0/Connector/R2020b\"],\"version\":\"1.0\"}"
  Neuron(Array) : Subsystem
      settings: PortSchema="{\"entries\":[{\"content\":{\"headerSize\":26,\"margin\":15,\"minimumSpacing\":25,\"sides\":[{\"content\":{},\"type\":\"ConnectorPlacement.EquallySpacedRectSide\",\"uuid\":\"08b5c2e0-5e4b-4108-9213-5cb3cfbc2fc7\"},{\"content\":{\"side\":\"RIGHT\"},\"type\":\"ConnectorPlacement.EquallySpacedRectSide\",\"uuid\":\"cef344b6-f3e5-417a-912f-da0044eb54ca\"},{\"content\":{\"connectorIds\":[\"In2\",\"In1\",\"Out1\",\"Out3\",\"Out4\",\"Out2\"],\"side\":\"TOP\"},\"type\":\"ConnectorPlacement.EquallySpacedRectSide\",\"uuid\":\"0b83641f-e918-4d2c-8db0-09bb563129af\"},{\"content\":{\"side\":\"BOTTOM\"},\"type\":\"ConnectorPlacement.EquallySpacedRectSide\",\"uuid\":\"6ae96cad-0b7a-4da8-9cd6-bd52ee925b68\"}]},\"type\":\"ConnectorPlacement.EquallySpacedConnector\",\"uuid\":\"45bfd962-fc80-412c-925f-742c48c6b5c0\"}],\"packageUris\":[\"http://schema.mathworks.com/mf0/Connector/R2020b\"],\"version\":\"1.0\"}"
  Bus Element Out2 : Outport  PortName=DFSW(RC_FINAL)
  Bus Element Out1 : Outport  Port=2  PortName=RC PostSpiketoOuter
  wires:
  Neuron(Array)/4(RC_PostSpike) -> AXIBus/4(RC_PostSpike)
  AXIBus/4(RC PostSpiketoOuter) -> Bus Element Out1/1
  Neuron(Array)/3(Deacticated Final Synaptic Weight) -> AXIBus/3(Deacticated Final Synaptic Weight)
  AXIBus/5(DFSW(RC_FINAL)) -> Bus Element Out2/1
  Neuron(Array)/1(DSFW(RC)) -> AXIBus/2(DFSW(RC))
  MAster/1(OutBus) -> AXIBus/1(InBus)
  AXIBus/3(OutBus) -> MAster/4(InBus)
  Bus Element In1/1 -> MAster/3($Neural Info Init_MC)
  AXIBus/2($Neural Info_NA) -> Neuron(Array)/1($Neural Info_NA)
  Bus Element In2/1 -> MAster/2(NeuralCodedData)
  AXIBus/1(NeuralCodedData(Spike)_NA) -> Neuron(Array)/2(External Spike)
  Bus Element In3/1 -> MAster/1(RC PostSpike From Another MC2)

== system hodumaru/NeuralProcessingUnit/MiniColumn(Array)/MiniColumn2 ==
  Bus Element In3 : Inport  PortName=RC PoskSpike From another MC
  Bus Element In2 : Inport  Port=2  PortName=NeuralCodedData
  Bus Element In1 : Inport  Port=3  PortName=$Neural Info Init_MC
  AXIBus : Subsystem
      settings: PortSchema="{\"entries\":[{\"content\":{\"headerSize\":26,\"margin\":15,\"minimumSpacing\":25,\"sides\":[{\"content\":{},\"type\":\"ConnectorPlacement.EquallySpacedRectSide\",\"uuid\":\"08b5c2e0-5e4b-4108-9213-5cb3cfbc2fc7\"},{\"content\":{\"connectorIds\":[\"Out5\",\"Out6\"],\"side\":\"RIGHT\"},\"type\":\"ConnectorPlacement.EquallySpacedRectSide\",\"uuid\":\"cef344b6-f3e5-417a-912f-da0044eb54ca\"},{\"content\":{\"connectorIds\":[\"In1\",\"Out4\"],\"side\":\"TOP\"},\"type\":\"ConnectorPlacement.EquallySpacedRectSide\",\"uuid\":\"0b83641f-e918-4d2c-8db0-09bb563129af\"},{\"content\":{\"connectorIds\":[\"Out1\",\"Out2\",\"Out3\",\"In2\",\"In3\",\"In4\"],\"side\":\"BOTTOM\"},\"type\":\"ConnectorPlacement.EquallySpacedRectSide\",\"uuid\":\"19498b06-f260-4dc1-a094-027c00d8d906\"}]},\"type\":\"ConnectorPlacement.EquallySpacedConnector\",\"uuid\":\"45bfd962-fc80-412c-925f-742c48c6b5c0\"}],\"packageUris\":[\"http://schema.mathworks.com/mf0/Connector/R2020b\"],\"version\":\"1.0\"}"
  MAster : Subsystem
      settings: PortSchema="{\"entries\":[{\"content\":{\"headerSize\":26,\"margin\":15,\"minimumSpacing\":25,\"sides\":[{\"content\":{\"connectorIds\":[\"In1\",\"In2\"]},\"type\":\"ConnectorPlacement.EquallySpacedRectSide\",\"uuid\":\"08b5c2e0-5e4b-4108-9213-5cb3cfbc2fc7\"},{\"content\":{\"connectorIds\":[\"In3\"],\"side\":\"RIGHT\"},\"type\":\"ConnectorPlacement.EquallySpacedRectSide\",\"uuid\":\"cef344b6-f3e5-417a-912f-da0044eb54ca\"},{\"content\":{\"side\":\"TOP\"},\"type\":\"ConnectorPlacement.EquallySpacedRectSide\",\"uuid\":\"0b83641f-e918-4d2c-8db0-09bb563129af\"},{\"content\":{\"connectorIds\":[\"Out1\",\"In4\"],\"side\":\"BOTTOM\"},\"type\":\"ConnectorPlacement.EquallySpacedRectSide\",\"uuid\":\"1d0526f4-c594-4b80-8124-d3d48d90ce30\"}]},\"type\":\"ConnectorPlacement.EquallySpacedConnector\",\"uuid\":\"45bfd962-fc80-412c-925f-742c48c6b5c0\"}],\"packageUris\":[\"http://schema.mathworks.com/mf0/Connector/R2020b\"],\"version\":\"1.0\"}"
  Neuron(Array) : Subsystem
      settings: PortSchema="{\"entries\":[{\"content\":{\"headerSize\":26,\"margin\":15,\"minimumSpacing\":25,\"sides\":[{\"content\":{},\"type\":\"ConnectorPlacement.EquallySpacedRectSide\",\"uuid\":\"08b5c2e0-5e4b-4108-9213-5cb3cfbc2fc7\"},{\"content\":{\"side\":\"RIGHT\"},\"type\":\"ConnectorPlacement.EquallySpacedRectSide\",\"uuid\":\"cef344b6-f3e5-417a-912f-da0044eb54ca\"},{\"content\":{\"connectorIds\":[\"In3\",\"In2\",\"In1\",\"Out1\",\"Out3\",\"Out4\",\"Out2\"],\"side\":\"TOP\"},\"type\":\"ConnectorPlacement.EquallySpacedRectSide\",\"uuid\":\"0b83641f-e918-4d2c-8db0-09bb563129af\"},{\"content\":{\"side\":\"BOTTOM\"},\"type\":\"ConnectorPlacement.EquallySpacedRectSide\",\"uuid\":\"6ae96cad-0b7a-4da8-9cd6-bd52ee925b68\"}]},\"type\":\"ConnectorPlacement.EquallySpacedConnector\",\"uuid\":\"45bfd962-fc80-412c-925f-742c48c6b5c0\"}],\"packageUris\":[\"http://schema.mathworks.com/mf0/Connector/R2020b\"],\"version\":\"1.0\"}"
  Bus Element Out2 : Outport  PortName=DFSW(RC_FINAL)
  Bus Element Out1 : Outport  Port=2  PortName=RC PostSpiketoOuter
  wires:
  Neuron(Array)/4(RC_PostSpike) -> AXIBus/4(RC_PostSpike)
  AXIBus/5(RC PostSpiketoOuter) -> Bus Element Out1/1
  Neuron(Array)/3(Deacticated Final Synaptic Weight) -> AXIBus/3(Deacticated Final Synaptic Weight)
  AXIBus/6(DFSW(RC_FINAL)) -> Bus Element Out2/1
  Neuron(Array)/1(DSFW(RC)) -> AXIBus/2(DFSW(RC))
  MAster/1(OutBus) -> AXIBus/1(InBus)
  AXIBus/4(OutBus) -> MAster/4(InBus)
  Bus Element In1/1 -> MAster/3($Neural Info Init_MC)
  AXIBus/3($Neural Info_NA) -> Neuron(Array)/1($Neural Info_NA)
  Bus Element In2/1 -> MAster/1(NeuralCodedData)
  AXIBus/1(NeuralCodedData(Spike)_NA) -> Neuron(Array)/3(External Spike)
  Bus Element In3/1 -> MAster/2(RC PoskSpike From another MC)
  AXIBus/2(RC PostSpike from another MC) -> Neuron(Array)/2(External Spike2)

== system hodumaru/NeuralProcessingUnit/MiniColumn(Array)/RichClubMemory(MCNI) ==
  Bus Element In1 : Inport  PortName=InBus
  Bus Element Out1 : Outport  PortName=OutBus

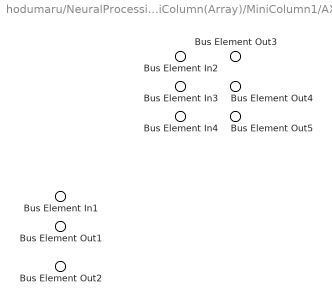
== system hodumaru/NeuralProcessingUnit/MiniColumn(Array)/MiniColumn1/AXIBus ==
  Bus Element In4 : Inport  PortName=InBus
  Bus Element In3 : Inport  Port=2  PortName=DFSW(RC)
  Bus Element In2 : Inport  Port=3  PortName=Deacticated Final Synaptic Weight
  Bus Element In1 : Inport  Port=4  PortName=RC_PostSpike
  Bus Element Out5 : Outport  PortName=NeuralCodedData(Spike)_NA
  Bus Element Out4 : Outport  Port=2  PortName=$Neural Info_NA
  Bus Element Out3 : Outport  Port=3  PortName=OutBus
  Bus Element Out1 : Outport  Port=4  PortName=RC PostSpiketoOuter
  Bus Element Out2 : Outport  Port=5  PortName=DFSW(RC_FINAL)

== system hodumaru/NeuralProcessingUnit/MiniColumn(Array)/MiniColumn1/MAster ==
  Bus Element In4 : Inport  PortName=RC PostSpike From Another MC2
  Bus Element In3 : Inport  Port=2  PortName=NeuralCodedData
  Bus Element In2 : Inport  Port=3  PortName=$Neural Info Init_MC
  Bus Element In1 : Inport  Port=4  PortName=InBus
  Bus Element Out1 : Outport  PortName=OutBus

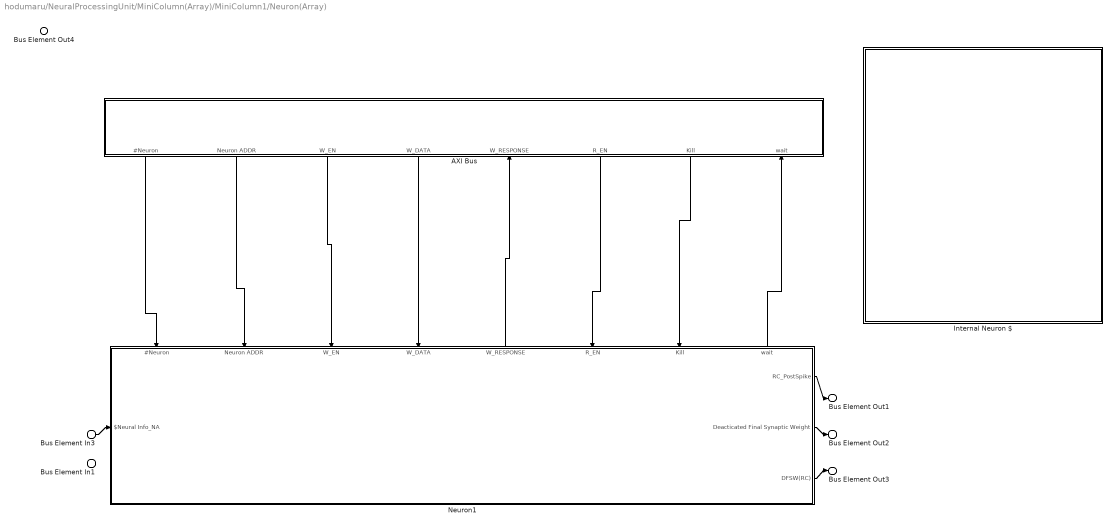
== system hodumaru/NeuralProcessingUnit/MiniColumn(Array)/MiniColumn1/Neuron(Array) ==
  Bus Element In3 : Inport  PortName=$Neural Info_NA
  Bus Element In1 : Inport  Port=2  PortName=External Spike
  AXI Bus : Subsystem
      settings: PortSchema="{\"entries\":[{\"content\":{\"headerSize\":26,\"margin\":15,\"minimumSpacing\":25,\"sides\":[{\"content\":{},\"type\":\"ConnectorPlacement.EquallySpacedRectSide\",\"uuid\":\"31e20200-2cb1-4382-9155-e0d85eeb6756\"},{\"content\":{\"side\":\"RIGHT\"},\"type\":\"ConnectorPlacement.EquallySpacedRectSide\",\"uuid\":\"e7a9e024-b9ad-4463-a43b-85143ff39b21\"},{\"content\":{\"side\":\"TOP\"},\"type\":\"ConnectorPlacement.EquallySpacedRectSide\",\"uuid\":\"8c8eb66f-8faf-4222-8ab7-6c33983befa5\"},{\"content\":{\"connectorIds\":[\"Out1\",\"Out2\",\"Out5\",\"Out3\",\"In1\",\"Out4\",\"Out6\",\"In2\"],\"side\":\"BOTTOM\"},\"type\":\"ConnectorPlacement.EquallySpacedRectSide\",\"uuid\":\"f73b198c-468f-4e11-9ea5-9ce367016b93\"}]},\"type\":\"ConnectorPlacement.EquallySpacedConnector\",\"uuid\":\"7102759c-7f33-40ec-8288-a87a26b0547f\"}],\"packageUris\":[\"http://schema.mathworks.com/mf0/Connector/R2020b\"],\"version\":\"1.0\"}"
  Internal Neuron $ : Subsystem
      settings: PortSchema="{\"entries\":[{\"content\":{\"headerSize\":26,\"margin\":15,\"minimumSpacing\":25,\"sides\":[{\"content\":{},\"type\":\"ConnectorPlacement.EquallySpacedRectSide\",\"uuid\":\"ebe87d50-b34c-4144-bb21-1b9f3994f650\"},{\"content\":{\"side\":\"RIGHT\"},\"type\":\"ConnectorPlacement.EquallySpacedRectSide\",\"uuid\":\"40dc9e4a-9138-4a47-a8ec-83303fc3d098\"},{\"content\":{\"side\":\"TOP\"},\"type\":\"ConnectorPlacement.EquallySpacedRectSide\",\"uuid\":\"74a947e4-452e-4cf6-9818-6ec720a0f546\"}]},\"type\":\"ConnectorPlacement.EquallySpacedConnector\",\"uuid\":\"10440d1f-8be4-47e4-a65a-b886e6188624\"}],\"packageUris\":[\"http://schema.mathworks.com/mf0/Connector/R2020b\"],\"version\":\"1.0\"}"
  Neuron1 : Subsystem
      settings: PortSchema="{\"entries\":[{\"content\":{\"headerSize\":26,\"margin\":15,\"minimumSpacing\":25,\"sides\":[{\"content\":{\"connectorIds\":[\"In7\"]},\"type\":\"ConnectorPlacement.EquallySpacedRectSide\",\"uuid\":\"e1193ddb-de85-49ee-b30a-e55681754550\"},{\"content\":{\"connectorIds\":[\"Out3\",\"Out4\",\"Out5\"],\"side\":\"RIGHT\"},\"type\":\"ConnectorPlacement.EquallySpacedRectSide\",\"uuid\":\"3d2e57d6-b7db-4720-9f64-4714c16315e3\"},{\"content\":{\"connectorIds\":[\"In1\",\"In2\",\"In5\",\"In3\",\"Out2\",\"In4\",\"In6\",\"Out1\"],\"side\":\"TOP\"},\"type\":\"ConnectorPlacement.EquallySpacedRectSide\",\"uuid\":\"c930f0e4-cc2e-4c20-ac5c-7cac1a35adac\"}]},\"type\":\"ConnectorPlacement.EquallySpacedConnector\",\"uuid\":\"5bed04ea-4742-42a3-b0a3-c412c3316964\"}],\"packageUris\":[\"http://schema.mathworks.com/mf0/Connector/R2020b\"],\"version\":\"1.0\"}"
  Bus Element Out4 : Outport  PortName=DSFW(RC)
  Bus Element Out3 : Outport  Port=2  PortName=DFSW(RC)
  Bus Element Out2 : Outport  Port=3  PortName=Deacticated Final Synaptic Weight
  Bus Element Out1 : Outport  Port=4  PortName=RC_PostSpike
  wires:
  Bus Element In3/1 -> Neuron1/7($Neural Info_NA)
  Neuron1/3(RC_PostSpike) -> Bus Element Out1/1
  Neuron1/4(Deacticated Final Synaptic Weight) -> Bus Element Out2/1
  Neuron1/5(DFSW(RC)) -> Bus Element Out3/1
  AXI Bus/5(W_EN) -> Neuron1/5(W_EN)
  Neuron1/2(W_RESPONSE) -> AXI Bus/1(W_RESPONSE)
  AXI Bus/4(R_EN) -> Neuron1/4(R_EN)
  AXI Bus/3(W_DATA) -> Neuron1/3(W_DATA)
  AXI Bus/2(Neuron ADDR) -> Neuron1/2(Neuron ADDR)
  AXI Bus/1(#Neuron) -> Neuron1/1(#Neuron)
  AXI Bus/6(Kill) -> Neuron1/6(Kill)
  Neuron1/1(wait) -> AXI Bus/2(wait)

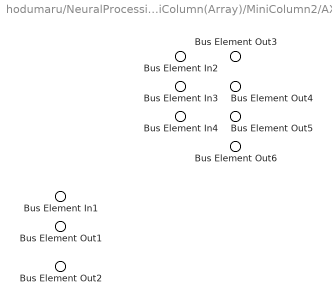
== system hodumaru/NeuralProcessingUnit/MiniColumn(Array)/MiniColumn2/AXIBus ==
  Bus Element In4 : Inport  PortName=InBus
  Bus Element In3 : Inport  Port=2  PortName=DFSW(RC)
  Bus Element In2 : Inport  Port=3  PortName=Deacticated Final Synaptic Weight
  Bus Element In1 : Inport  Port=4  PortName=RC_PostSpike
  Bus Element Out5 : Outport  PortName=NeuralCodedData(Spike)_NA
  Bus Element Out6 : Outport  Port=2  PortName=RC PostSpike from another MC
  Bus Element Out4 : Outport  Port=3  PortName=$Neural Info_NA
  Bus Element Out3 : Outport  Port=4  PortName=OutBus
  Bus Element Out1 : Outport  Port=5  PortName=RC PostSpiketoOuter
  Bus Element Out2 : Outport  Port=6  PortName=DFSW(RC_FINAL)

== system hodumaru/NeuralProcessingUnit/MiniColumn(Array)/MiniColumn2/MAster ==
  Bus Element In3 : Inport  PortName=NeuralCodedData
  Bus Element In4 : Inport  Port=2  PortName=RC PoskSpike From another MC
  Bus Element In2 : Inport  Port=3  PortName=$Neural Info Init_MC
  Bus Element In1 : Inport  Port=4  PortName=InBus
  Bus Element Out1 : Outport  PortName=OutBus

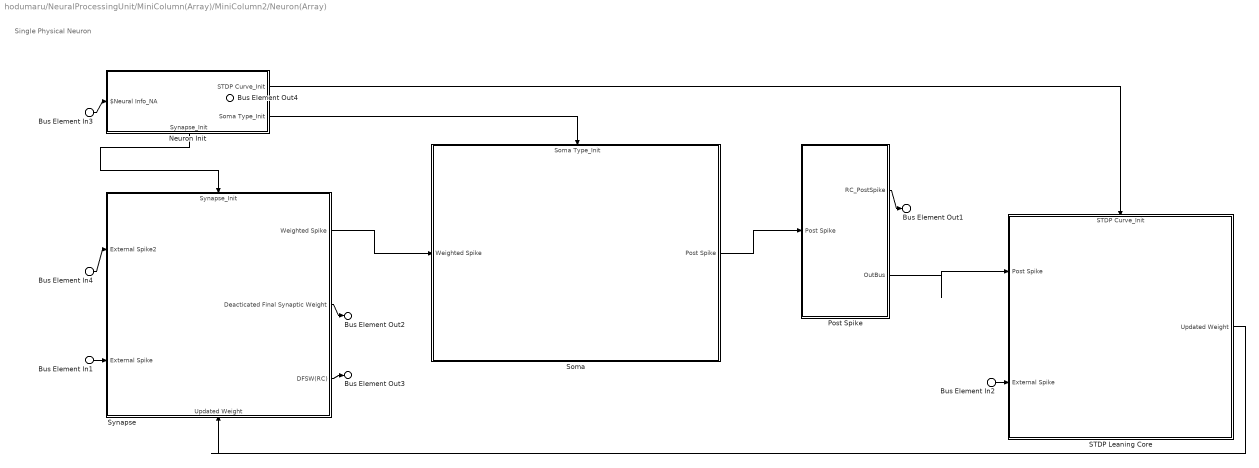
== system hodumaru/NeuralProcessingUnit/MiniColumn(Array)/MiniColumn2/Neuron(Array) ==
  note: Single Physical Neuron
  Bus Element In3 : Inport  PortName=$Neural Info_NA
  Bus Element In4 : Inport  Port=2  PortName=External Spike2
  Bus Element In1 : Inport  Port=3  PortName=External Spike
  Bus Element In2 : Inport  Port=3  PortName=External Spike
  Neuron Init : Subsystem
      settings: PortSchema="{\"entries\":[{\"content\":{\"headerSize\":26,\"margin\":15,\"minimumSpacing\":25,\"sides\":[{\"content\":{\"connectorIds\":[\"In1\"]},\"type\":\"ConnectorPlacement.EquallySpacedRectSide\",\"uuid\":\"31e20200-2cb1-4382-9155-e0d85eeb6756\"},{\"content\":{\"connectorIds\":[\"Out1\",\"Out2\"],\"side\":\"RIGHT\"},\"type\":\"ConnectorPlacement.EquallySpacedRectSide\",\"uuid\":\"e7a9e024-b9ad-4463-a43b-85143ff39b21\"},{\"content\":{\"side\":\"TOP\"},\"type\":\"ConnectorPlacement.EquallySpacedRectSide\",\"uuid\":\"8c8eb66f-8faf-4222-8ab7-6c33983befa5\"},{\"content\":{\"connectorIds\":[\"Out3\"],\"side\":\"BOTTOM\"},\"type\":\"ConnectorPlacement.EquallySpacedRectSide\",\"uuid\":\"0439fc03-e407-47dd-9672-15c503cc2279\"}]},\"type\":\"ConnectorPlacement.EquallySpacedConnector\",\"uuid\":\"7102759c-7f33-40ec-8288-a87a26b0547f\"}],\"packageUris\":[\"http://schema.mathworks.com/mf0/Connector/R2020b\"],\"version\":\"1.0\"}"
  Post Spike : Subsystem
      settings: PortSchema="{\"entries\":[{\"content\":{\"headerSize\":26,\"margin\":15,\"minimumSpacing\":25,\"sides\":[{\"content\":{\"connectorIds\":[\"In1\"]},\"type\":\"ConnectorPlacement.EquallySpacedRectSide\",\"uuid\":\"31e20200-2cb1-4382-9155-e0d85eeb6756\"},{\"content\":{\"connectorIds\":[\"Out1\",\"Out2\"],\"side\":\"RIGHT\"},\"type\":\"ConnectorPlacement.EquallySpacedRectSide\",\"uuid\":\"e7a9e024-b9ad-4463-a43b-85143ff39b21\"},{\"content\":{\"side\":\"TOP\"},\"type\":\"ConnectorPlacement.EquallySpacedRectSide\",\"uuid\":\"8c8eb66f-8faf-4222-8ab7-6c33983befa5\"}]},\"type\":\"ConnectorPlacement.EquallySpacedConnector\",\"uuid\":\"7102759c-7f33-40ec-8288-a87a26b0547f\"}],\"packageUris\":[\"http://schema.mathworks.com/mf0/Connector/R2020b\"],\"version\":\"1.0\"}"
  STDP Leaning Core : Subsystem
      settings: PortSchema="{\"entries\":[{\"content\":{\"headerSize\":26,\"margin\":15,\"minimumSpacing\":25,\"sides\":[{\"content\":{\"connectorIds\":[\"In1\",\"In3\"]},\"type\":\"ConnectorPlacement.EquallySpacedRectSide\",\"uuid\":\"08b5c2e0-5e4b-4108-9213-5cb3cfbc2fc7\"},{\"content\":{\"connectorIds\":[\"Out1\"],\"side\":\"RIGHT\"},\"type\":\"ConnectorPlacement.EquallySpacedRectSide\",\"uuid\":\"cef344b6-f3e5-417a-912f-da0044eb54ca\"},{\"content\":{\"connectorIds\":[\"In2\"],\"side\":\"TOP\"},\"type\":\"ConnectorPlacement.EquallySpacedRectSide\",\"uuid\":\"0b83641f-e918-4d2c-8db0-09bb563129af\"}]},\"type\":\"ConnectorPlacement.EquallySpacedConnector\",\"uuid\":\"45bfd962-fc80-412c-925f-742c48c6b5c0\"}],\"packageUris\":[\"http://schema.mathworks.com/mf0/Connector/R2020b\"],\"version\":\"1.0\"}"
  Soma : Subsystem
      settings: PortSchema="{\"entries\":[{\"content\":{\"headerSize\":26,\"margin\":15,\"minimumSpacing\":25,\"sides\":[{\"content\":{\"connectorIds\":[\"In2\"]},\"type\":\"ConnectorPlacement.EquallySpacedRectSide\",\"uuid\":\"08b5c2e0-5e4b-4108-9213-5cb3cfbc2fc7\"},{\"content\":{\"connectorIds\":[\"Out1\"],\"side\":\"RIGHT\"},\"type\":\"ConnectorPlacement.EquallySpacedRectSide\",\"uuid\":\"cef344b6-f3e5-417a-912f-da0044eb54ca\"},{\"content\":{\"connectorIds\":[\"In1\"],\"side\":\"TOP\"},\"type\":\"ConnectorPlacement.EquallySpacedRectSide\",\"uuid\":\"0b83641f-e918-4d2c-8db0-09bb563129af\"}]},\"type\":\"ConnectorPlacement.EquallySpacedConnector\",\"uuid\":\"45bfd962-fc80-412c-925f-742c48c6b5c0\"}],\"packageUris\":[\"http://schema.mathworks.com/mf0/Connector/R2020b\"],\"version\":\"1.0\"}"
  Synapse : Subsystem
      settings: PortSchema="{\"entries\":[{\"content\":{\"headerSize\":26,\"margin\":15,\"minimumSpacing\":25,\"sides\":[{\"content\":{\"connectorIds\":[\"In1\",\"In4\"]},\"type\":\"ConnectorPlacement.EquallySpacedRectSide\",\"uuid\":\"08b5c2e0-5e4b-4108-9213-5cb3cfbc2fc7\"},{\"content\":{\"connectorIds\":[\"Out1\",\"Out2\",\"Out3\"],\"side\":\"RIGHT\"},\"type\":\"ConnectorPlacement.EquallySpacedRectSide\",\"uuid\":\"cef344b6-f3e5-417a-912f-da0044eb54ca\"},{\"content\":{\"connectorIds\":[\"In2\"],\"side\":\"TOP\"},\"type\":\"ConnectorPlacement.EquallySpacedRectSide\",\"uuid\":\"0b83641f-e918-4d2c-8db0-09bb563129af\"},{\"content\":{\"connectorIds\":[\"In3\"],\"side\":\"BOTTOM\"},\"type\":\"ConnectorPlacement.EquallySpacedRectSide\",\"uuid\":\"115d5a97-31cb-4c10-ac03-233646a622a9\"}]},\"type\":\"ConnectorPlacement.EquallySpacedConnector\",\"uuid\":\"45bfd962-fc80-412c-925f-742c48c6b5c0\"}],\"packageUris\":[\"http://schema.mathworks.com/mf0/Connector/R2020b\"],\"version\":\"1.0\"}"
  Bus Element Out4 : Outport  PortName=DSFW(RC)
  Bus Element Out3 : Outport  Port=2  PortName=DFSW(RC)
  Bus Element Out2 : Outport  Port=3  PortName=Deacticated Final Synaptic Weight
  Bus Element Out1 : Outport  Port=4  PortName=RC_PostSpike
  wires:
  Bus Element In1/1 -> Synapse/4(External Spike)
  Synapse/1(Weighted Spike) -> Soma/2(Weighted Spike)
  Bus Element In2/1 -> STDP Leaning Core/3(External Spike)
  STDP Leaning Core/1(Updated Weight) -> Synapse/3(Updated Weight)
  Synapse/2(Deacticated Final Synaptic Weight) -> Bus Element Out2/1
  Synapse/3(DFSW(RC)) -> Bus Element Out3/1
  Neuron Init/3(Synapse_Init) -> Synapse/2(Synapse_Init)
  Bus Element In3/1 -> Neuron Init/1($Neural Info_NA)
  Neuron Init/2(Soma Type_Init) -> Soma/1(Soma Type_Init)
  Neuron Init/1(STDP Curve_Init) -> STDP Leaning Core/2(STDP Curve_Init)
  Soma/1(Post Spike) -> Post Spike/1(Post Spike)
  Post Spike/1(RC_PostSpike) -> Bus Element Out1/1
  Post Spike/2(OutBus) -> STDP Leaning Core/1(Post Spike)
  Bus Element In4/1 -> Synapse/1(External Spike2)

== system hodumaru/NeuralProcessingUnit/MiniColumn(Array)/MiniColumn1/Neuron(Array)/AXI Bus ==
  Bus Element In1 : Inport  PortName=W_RESPONSE
  Bus Element In2 : Inport  Port=2  PortName=wait
  Bus Element Out1 : Outport  PortName=#Neuron
  Bus Element Out5 : Outport  Port=2  PortName=Neuron ADDR
  Bus Element Out4 : Outport  Port=3  PortName=W_DATA
  Bus Element Out3 : Outport  Port=4  PortName=R_EN
  Bus Element Out2 : Outport  Port=5  PortName=W_EN
  Bus Element Out6 : Outport  Port=6  PortName=Kill

== system hodumaru/NeuralProcessingUnit/MiniColumn(Array)/MiniColumn1/Neuron(Array)/Internal Neuron $ ==
